simulink library "csthl20_lib"  (R2022a)
settings: Solver=VariableStepAuto  StartTime=0.0  StopTime=10.0  RelTol=1e-3
undefined symbols (not defined in the file or in its folder): alpha_vec_Cn0, b_ref, beta_vec_Cn0, Clbeta, Clda, Clddf, Cldr, Clp, Clr, Cm0, Cmda, Cmde, Cmdfn, Cmdfp, Cmdr, Cmq, Cn0, Cnda, Cnddf, Cndr, Cnp, Cnr, CX0, CXda, CXddf, CXde, CXdfn, CXdfp, CXdr, CYbeta, CYda, CYddf, CYdr, CZ0, CZda, CZde, CZdfn, CZdfp, CZdr, d_ref, mass, x_cg, x_ref
libraries: aerolibasang x3, aerolibconvert2 x2, shared6dof x1, aerolibatmos2 x1, aerolibobsolete x1, aerolibadyn x1
settings Model: Creator=The MathWorks, Inc.  LastModifiedBy=The MathWorks, Inc.
settings SolverCC: AlgebraicLoopSolver=TrustRegion
settings DataIOCC: ReturnWorkspaceOutputs=off
settings DebuggingCC: UnconnectedInputMsg=warning  UnconnectedOutputMsg=warning  UnconnectedLineMsg=warning  SFMachineParentedDataDiag=warning  ArithmeticOperatorsInVariantConditions=warning
settings SFSimCC: SimUseLocalCustomCode=off  CustomCodeUndefinedFunction=UseInterfaceOnly
settings RTWCC: RTWUseLocalCustomCode=off

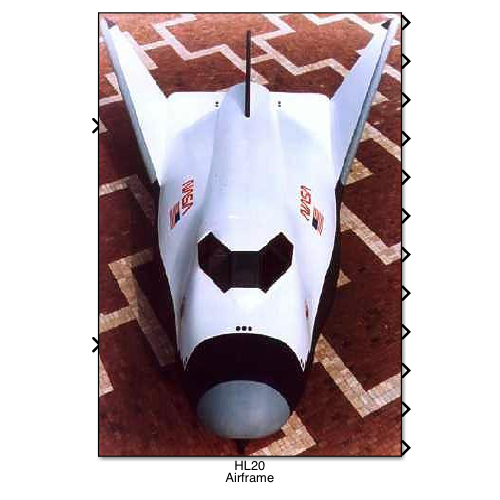
[thumbnail: Simulink's stored preview of the top-level diagram]
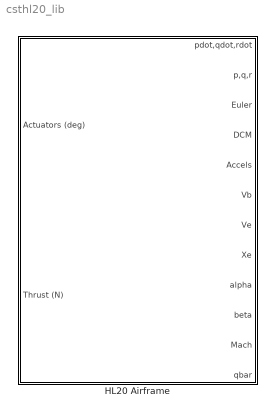
== system csthl20_lib ==
  HL20 Airframe : Subsystem
      mask Display: image('aeroblk_HL20pic.jpg')

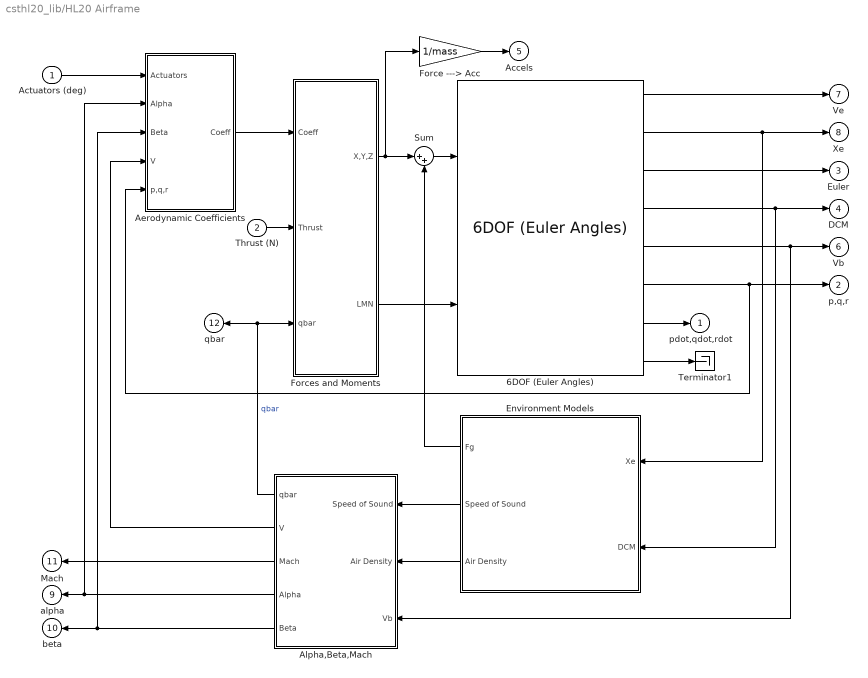
== system csthl20_lib/HL20 Airframe ==
  Actuators (deg) : Inport  Unit=deg
  Thrust (N) : Inport  Port=2  Unit=N
  6DOF (Euler Angles) : shared6dof/6DOF (Euler Angles)  units=Metric (MKS)  mtype=Fixed  rep=Euler Angles  xme_0=xme_0  Vm_0=Vmw  eul_0=Euler_0  pm_0=pm_0  mass_0=mass  mass_e=0.5  mass_f=2.0  inertia=Inertia  inertia_e=eye(3)  inertia_f=2*eye(3)  k_quat=1.0  vre_flag=on  abi_flag=off  aMode=aMode  xme_statename=''  Vm_statename=''  eul_statename=''  quat_statename=''  pm_statename=''  mass_statename=''
      settings: SourceProductBaseCode=AE,PW,DR,MT,VE
  Aerodynamic Coefficients : Subsystem
  Alpha,Beta,Mach : Subsystem
  Environment Models : Subsystem
  Force ---> Acc : Gain  Gain=1/mass  SaturateOnIntegerOverflow=on  OutDataTypeStr=Inherit: Same as input  ParamDataTypeStr=Inherit: Same as input
  Forces and Moments : Subsystem
  Sum : Sum  Inputs=|++  InputSameDT=on  SaturateOnIntegerOverflow=on  OutDataTypeStr=Inherit: Same as first input
  Terminator1 : Terminator
  pdot,qdot,rdot : Outport  Unit=rad/s^2  InitialOutput=0  VectorParamsAs1DForOutWhenUnconnected=off
  p,q,r : Outport  Port=2  Unit=rad/second  InitialOutput=0  VectorParamsAs1DForOutWhenUnconnected=off
  Euler : Outport  Port=3  Unit=rad  InitialOutput=0  VectorParamsAs1DForOutWhenUnconnected=off
  DCM : Outport  Port=4  InitialOutput=0  VectorParamsAs1DForOutWhenUnconnected=off
  Accels : Outport  Port=5  Unit=m/s^2  InitialOutput=0  VectorParamsAs1DForOutWhenUnconnected=off
  Vb : Outport  Port=6  Unit=m/second  InitialOutput=0  VectorParamsAs1DForOutWhenUnconnected=off
  Ve : Outport  Port=7  Unit=m/second  InitialOutput=0  VectorParamsAs1DForOutWhenUnconnected=off
  Xe : Outport  Port=8  Unit=meter  InitialOutput=0  VectorParamsAs1DForOutWhenUnconnected=off
  alpha : Outport  Port=9  Unit=rad  InitialOutput=0  VectorParamsAs1DForOutWhenUnconnected=off
  beta : Outport  Port=10  Unit=rad  InitialOutput=0  VectorParamsAs1DForOutWhenUnconnected=off
  Mach : Outport  Port=11  InitialOutput=0  VectorParamsAs1DForOutWhenUnconnected=off
  qbar : Outport  Port=12  Unit=Pa  InitialOutput=0  VectorParamsAs1DForOutWhenUnconnected=off
  wires:
  Alpha,Beta,Mach/5(Beta) -> beta/1, Aerodynamic Coefficients/3(Beta)
  Alpha,Beta,Mach/3(Mach) -> Mach/1
  Alpha,Beta,Mach/2(V) -> Aerodynamic Coefficients/4(V)
  Actuators (deg)/1 -> Aerodynamic Coefficients/1(Actuators)
  Force ---> Acc/1 -> Accels/1
  Environment Models/1(Fg) -> Sum/2
  Sum/1 -> 6DOF (Euler Angles)/1
  Forces and Moments/1(X,Y,Z) -> Sum/1, Force ---> Acc/1
  Alpha,Beta,Mach/1(qbar) -> qbar/1, Forces and Moments/3(qbar)  "qbar"
  Forces and Moments/2(LMN) -> 6DOF (Euler Angles)/2
  Environment Models/3(Air Density) -> Alpha,Beta,Mach/2(Air Density)
  Environment Models/2(Speed of Sound) -> Alpha,Beta,Mach/1(Speed of Sound)
  6DOF (Euler Angles)/5 -> Vb/1, Alpha,Beta,Mach/3(Vb)
  Aerodynamic Coefficients/1(Coeff) -> Forces and Moments/1(Coeff)
  Alpha,Beta,Mach/4(Alpha) -> alpha/1, Aerodynamic Coefficients/2(Alpha)
  6DOF (Euler Angles)/3 -> Euler/1
  6DOF (Euler Angles)/4 -> Environment Models/2(DCM), DCM/1
  6DOF (Euler Angles)/7 -> pdot,qdot,rdot/1
  Thrust (N)/1 -> Forces and Moments/2(Thrust)
  6DOF (Euler Angles)/6 -> p,q,r/1, Aerodynamic Coefficients/5(p,q,r)
  6DOF (Euler Angles)/2 -> Xe/1, Environment Models/1(Xe)
  6DOF (Euler Angles)/1 -> Ve/1
  6DOF (Euler Angles)/8 -> Terminator1/1

== system csthl20_lib/HL20 Airframe/Aerodynamic Coefficients ==
  Actuators : Inport
  Alpha : Inport  Port=2
  Beta : Inport  Port=3
  V : Inport  Port=4
  p,q,r : Inport  Port=5
  Actuator Increments : Subsystem
  Body Rate Damping : Subsystem
  Datum Coefficients : Subsystem
  Sum1 : Sum  Inputs=+++  InputSameDT=on  SaturateOnIntegerOverflow=on  OutDataTypeStr=Inherit: Same as first input
  alpha_rad : aerolibconvert2/Angle Conversion  IU=rad  OU=deg
  beta_rad : aerolibconvert2/Angle Conversion  IU=rad  OU=deg
  Coeff : Outport  VectorParamsAs1DForOutWhenUnconnected=off
  wires:
  Alpha/1 -> alpha_rad/1
  Beta/1 -> beta_rad/1
  alpha_rad/1 -> Body Rate Damping/3(Alpha), Datum Coefficients/1(Alpha), Actuator Increments/1(Alpha)
  p,q,r/1 -> Body Rate Damping/2(p,q,r)
  Actuators/1 -> Actuator Increments/3("Actuator Deflections ")
  Sum1/1 -> Coeff/1
  Datum Coefficients/1(cl) -> Sum1/2
  beta_rad/1 -> Datum Coefficients/2(Beta), Actuator Increments/2(Beta)
  V/1 -> Body Rate Damping/1(V)
  Body Rate Damping/1(cl) -> Sum1/1
  Actuator Increments/1(cl) -> Sum1/3

== system csthl20_lib/HL20 Airframe/Alpha,Beta,Mach ==
  note: TODO: clean up interface
  Speed of Sound : Inport
  Air Density : Inport  Port=2
  Vb : Inport  Port=3  PortDimensions=3
  Dynamic Pressure : aerolibasang/Dynamic Pressure
  "Incidence, Sideslip, & Airspeed" : aerolibasang/Incidence, Sideslip, & Airspeed
  Mach Number : aerolibasang/Mach Number
      settings: SourceProductBaseCode=AE
  qbar : Outport  Unit=Pa  InitialOutput=0  VectorParamsAs1DForOutWhenUnconnected=off
  V : Outport  Port=2  Unit=m/s  VectorParamsAs1DForOutWhenUnconnected=off
  Mach : Outport  Port=3  VectorParamsAs1DForOutWhenUnconnected=off
  Alpha : Outport  Port=4  Unit=rad  VectorParamsAs1DForOutWhenUnconnected=off
  Beta : Outport  Port=5  Unit=rad  VectorParamsAs1DForOutWhenUnconnected=off
  wires:
  Air Density/1 -> Dynamic Pressure/2
  Speed of Sound/1 -> Mach Number/2
  "Incidence, Sideslip, & Airspeed"/2 -> Beta/1  "Beta"
  "Incidence, Sideslip, & Airspeed"/3 -> V/1  "V"
  Vb/1 -> "Incidence, Sideslip, & Airspeed"/1, Mach Number/1, Dynamic Pressure/1
  "Incidence, Sideslip, & Airspeed"/1 -> Alpha/1  "Alpha"
  Mach Number/1 -> Mach/1  "Mach"
  Dynamic Pressure/1 -> qbar/1  "qbar"

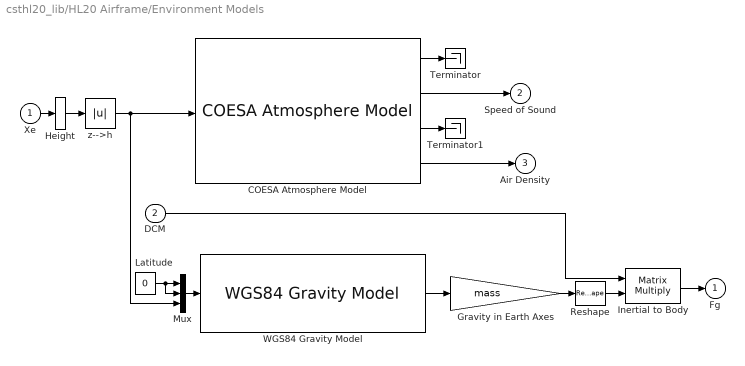
== system csthl20_lib/HL20 Airframe/Environment Models ==
  Xe : Inport  Unit=meter  PortDimensions=3
  DCM : Inport  Port=2
  COESA Atmosphere Model : aerolibatmos2/COESA Atmosphere Model  units=Metric (MKS)  spec=1976 COESA-extended U.S. Standard Atmosphere  model=Profile  profile_var=High temperature  profile_percent=10%  profile_alt=5 km (16404 ft)  envelope_var=High temperature  envelope_percent=1%  action=None
  Gravity in Earth Axes : Gain  Gain=mass  SaturateOnIntegerOverflow=on  OutDataTypeStr=Inherit: Same as input  ParamDataTypeStr=Inherit: Same as input
  Height : Selector  InputPortWidth=3  IndexOptions=Index vector (dialog)  Indices=[3]  OutputSizes=1
  Inertial to Body : Product  Multiplication=Matrix(*)  InputSameDT=on  SaturateOnIntegerOverflow=on  OutDataTypeStr=Inherit: Same as first input
  Latitude : Constant  Value=0
  Mux : Mux  Inputs=3
  Reshape : Reshape
  Terminator : Terminator
  Terminator1 : Terminator
  "WGS84 Gravity Model " : aerolibobsolete/WGS84 Gravity Model   model=WGS84 Taylor Series  units=Metric (MKS)  no_atmos=on  precessing=on  jd_loc=off  month=October  day=10  year=2004  no_centrifugal=on  action=None
      settings: SourceProductBaseCode=AE
  z-->h : Abs
  Fg : Outport  Unit=N  InitialOutput=0  VectorParamsAs1DForOutWhenUnconnected=off
  Speed of Sound : Outport  Port=2  Unit=m/second  InitialOutput=0  VectorParamsAs1DForOutWhenUnconnected=off
  Air Density : Outport  Port=3  Unit=kg/m^3  InitialOutput=0  VectorParamsAs1DForOutWhenUnconnected=off
  wires:
  "WGS84 Gravity Model "/1 -> Gravity in Earth Axes/1
  Inertial to Body/1 -> Fg/1
  DCM/1 -> Inertial to Body/1
  Gravity in Earth Axes/1 -> Reshape/1
  Latitude/1 -> Mux/1, Mux/2
  Xe/1 -> Height/1
  Height/1 -> z-->h/1
  COESA Atmosphere Model/1 -> Terminator/1
  COESA Atmosphere Model/3 -> Terminator1/1
  COESA Atmosphere Model/2 -> Speed of Sound/1
  COESA Atmosphere Model/4 -> Air Density/1
  z-->h/1 -> COESA Atmosphere Model/1, Mux/3
  Mux/1 -> "WGS84 Gravity Model "/1
  Reshape/1 -> Inertial to Body/2

== system csthl20_lib/HL20 Airframe/Forces and Moments ==
  Coeff : Inport
  Thrust : Inport  Port=2  Unit=N
  qbar : Inport  Port=3  Unit=Pa
  Aerodynamic Forces and Moments : aerolibadyn/Aerodynamic Forces and Moments   inputAxes=Body  outputForceAxes=Body  outputMomentAxes=Body  S=S_ref  b=b_ref  cbar=d_ref
  Center of Gravity : Constant  Value=[-x_cg 0 0]
  Center of Pressure : Constant  Value=[- x_ref 0 0]
  Sum : Sum  Inputs=++|  InputSameDT=on  SaturateOnIntegerOverflow=on  OutDataTypeStr=Inherit: Same as first input
  X,Y,Z : Outport  Unit=N  InitialOutput=0  VectorParamsAs1DForOutWhenUnconnected=off
  LMN : Outport  Port=2  Unit=N*m  InitialOutput=0  VectorParamsAs1DForOutWhenUnconnected=off
  wires:
  Coeff/1 -> Aerodynamic Forces and Moments/1
  qbar/1 -> Aerodynamic Forces and Moments/2
  Thrust/1 -> Sum/1
  Sum/1 -> X,Y,Z/1
  Aerodynamic Forces and Moments/2 -> LMN/1
  Aerodynamic Forces and Moments/1 -> Sum/2
  Center of Gravity/1 -> Aerodynamic Forces and Moments/3
  Center of Pressure/1 -> Aerodynamic Forces and Moments/4

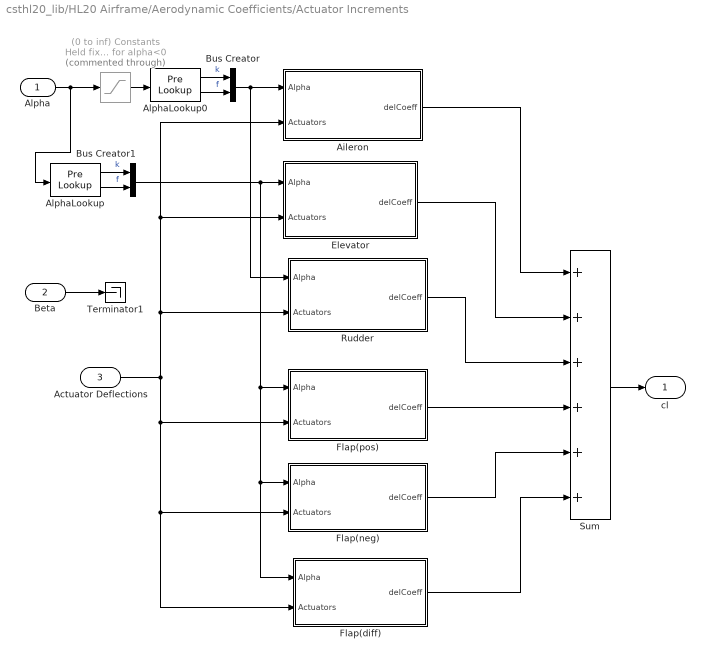
== system csthl20_lib/HL20 Airframe/Aerodynamic Coefficients/Actuator Increments ==
  Alpha : Inport
  Beta : Inport  Port=2
  "Actuator Deflections " : Inport  Port=3
  (0 to inf) Constants Held fixed for alpha<0 : Saturate  Commented=through  UpperLimit=inf  LowerLimit=0
  Aileron : Subsystem
  AlphaLookup : PreLookup  BreakpointsData=alpha_vec_0  BeginIndexSearchUsingPreviousIndexResult=on  ExtrapMethod=Linear
  AlphaLookup0 : PreLookup  BreakpointsData=alpha_vec_0  BeginIndexSearchUsingPreviousIndexResult=on  ExtrapMethod=Linear
  Bus Creator : BusCreator  Inputs=2
  Bus Creator1 : BusCreator  Inputs=2
  Elevator : Subsystem
  Flap(diff) : Subsystem
  Flap(neg) : Subsystem
  Flap(pos) : Subsystem
  Rudder : Subsystem
  Sum : Sum  Inputs=++++++  InputSameDT=on  SaturateOnIntegerOverflow=on  OutDataTypeStr=Inherit: Same as first input
  Terminator1 : Terminator
  cl : Outport  InitialOutput=0  VectorParamsAs1DForOutWhenUnconnected=off
  wires:
  Bus Creator/1 -> Aileron/1(Alpha), Rudder/1(Alpha)
  (0 to inf) Constants Held fixed for alpha<0/1 -> AlphaLookup0/1
  "Actuator Deflections "/1 -> Aileron/2(Actuators), Elevator/2(Actuators), Rudder/2(Actuators), Flap(pos)/2(Actuators), Flap(neg)/2(Actuators), Flap(diff)/2(Actuators)
  Alpha/1 -> (0 to inf) Constants Held fixed for alpha<0/1, AlphaLookup/1
  Beta/1 -> Terminator1/1
  Aileron/1(delCoeff) -> Sum/1
  Elevator/1(delCoeff) -> Sum/2
  Rudder/1(delCoeff) -> Sum/3
  Flap(pos)/1(delCoeff) -> Sum/4
  Flap(neg)/1(delCoeff) -> Sum/5
  Flap(diff)/1(delCoeff) -> Sum/6
  Sum/1 -> cl/1
  Bus Creator1/1 -> Flap(diff)/1(Alpha), Flap(neg)/1(Alpha), Flap(pos)/1(Alpha), Elevator/1(Alpha)
  AlphaLookup0/1 -> Bus Creator/1  "k"
  AlphaLookup0/2 -> Bus Creator/2  "f"
  AlphaLookup/1 -> Bus Creator1/1  "k"
  AlphaLookup/2 -> Bus Creator1/2  "f"

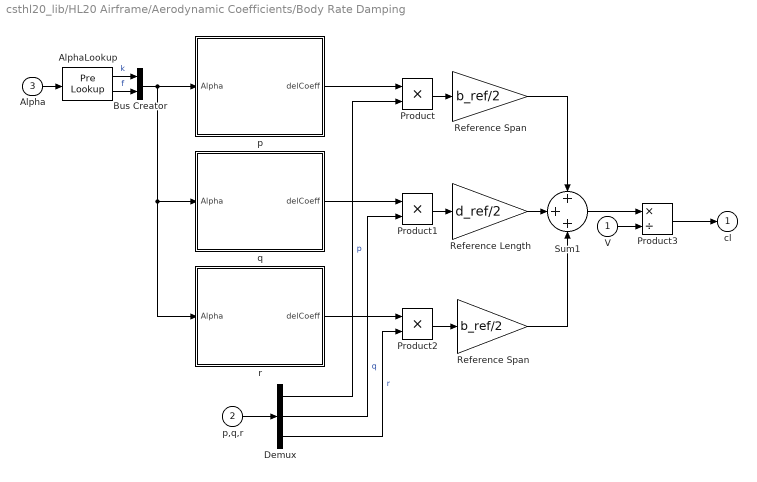
== system csthl20_lib/HL20 Airframe/Aerodynamic Coefficients/Body Rate Damping ==
  V : Inport
  p,q,r : Inport  Port=2
  Alpha : Inport  Port=3
  AlphaLookup : PreLookup  BreakpointsData=alpha_vec_damping  BeginIndexSearchUsingPreviousIndexResult=on  ExtrapMethod=Linear
  Bus Creator : BusCreator  Inputs=2
  Demux : Demux  Outputs=3
      settings: DisplayOption=none
  Product : Product  InputSameDT=on  SaturateOnIntegerOverflow=on  OutDataTypeStr=Inherit: Same as first input
  Product1 : Product  InputSameDT=on  SaturateOnIntegerOverflow=on  OutDataTypeStr=Inherit: Same as first input
  Product2 : Product  InputSameDT=on  SaturateOnIntegerOverflow=on  OutDataTypeStr=Inherit: Same as first input
  Product3 : Product  Inputs=*/  InputSameDT=on  SaturateOnIntegerOverflow=on  OutDataTypeStr=Inherit: Same as first input
  Reference Length : Gain  Gain=d_ref/2  SaturateOnIntegerOverflow=on  OutDataTypeStr=Inherit: Same as input  ParamDataTypeStr=Inherit: Same as input
  Reference Span : Gain  Gain=b_ref/2  SaturateOnIntegerOverflow=on  OutDataTypeStr=Inherit: Same as input  ParamDataTypeStr=Inherit: Same as input
  "Reference Span " : Gain  Gain=b_ref/2  SaturateOnIntegerOverflow=on  OutDataTypeStr=Inherit: Same as input  ParamDataTypeStr=Inherit: Same as input
  Sum1 : Sum  Inputs=+++  InputSameDT=on  SaturateOnIntegerOverflow=on  OutDataTypeStr=Inherit: Same as first input
  p : Subsystem
  q : Subsystem
  r : Subsystem
  cl : Outport  InitialOutput=0  VectorParamsAs1DForOutWhenUnconnected=off
  wires:
  Alpha/1 -> AlphaLookup/1
  p/1(delCoeff) -> Product/1
  q/1(delCoeff) -> Product1/1
  p,q,r/1 -> Demux/1
  Demux/1 -> Product/2  "p"
  Demux/2 -> Product1/2  "q"
  Demux/3 -> Product2/2  "r"
  Sum1/1 -> Product3/1
  V/1 -> Product3/2
  Product3/1 -> cl/1
  Product1/1 -> Reference Length/1
  Product2/1 -> "Reference Span "/1
  Product/1 -> Reference Span/1
  r/1(delCoeff) -> Product2/1
  Bus Creator/1 -> r/1(Alpha), q/1(Alpha), p/1(Alpha)
  Reference Length/1 -> Sum1/2
  Reference Span/1 -> Sum1/1
  "Reference Span "/1 -> Sum1/3
  AlphaLookup/1 -> Bus Creator/1  "k"
  AlphaLookup/2 -> Bus Creator/2  "f"

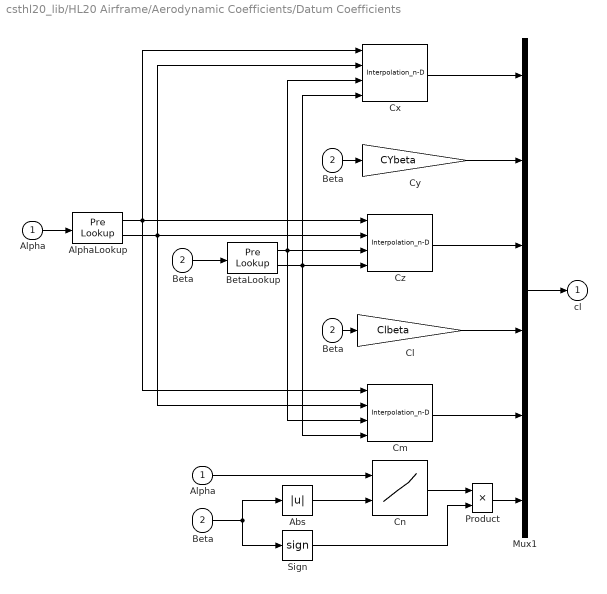
== system csthl20_lib/HL20 Airframe/Aerodynamic Coefficients/Datum Coefficients ==
  Alpha : Inport
  Beta : Inport  Port=2
  " Cn" : Lookup_n-D  BreakpointsForDimension1=alpha_vec_Cn0  BreakpointsForDimension2=beta_vec_Cn0  Table=Cn0  InternalRulePriority=Speed  RndMeth=Simplest
      settings: InputPortMap=u0,u1
  " Beta" : InportShadow  Port=2
  " Beta " : InportShadow  Port=2
  Abs : Abs
  "Alpha " : InportShadow
  AlphaLookup : PreLookup  BreakpointsData=alpha_vec_0  BeginIndexSearchUsingPreviousIndexResult=on  ExtrapMethod=Linear
  "Beta " : InportShadow  Port=2
  BetaLookup : PreLookup  BreakpointsData=beta_vec_0  BeginIndexSearchUsingPreviousIndexResult=on  ExtrapMethod=Linear
  Cl : Gain  Gain=Clbeta  SaturateOnIntegerOverflow=on  OutDataTypeStr=Inherit: Same as input  ParamDataTypeStr=Inherit: Same as input
  Cm : Interpolation_n-D  Table=Cm0'  RemoveProtectionIndex=on  SaturateOnIntegerOverflow=on
  Cx : Interpolation_n-D  Table=CX0'  RemoveProtectionIndex=on  SaturateOnIntegerOverflow=on
  Cy : Gain  Gain=CYbeta  SaturateOnIntegerOverflow=on  OutDataTypeStr=Inherit: Same as input  ParamDataTypeStr=Inherit: Same as input
  Cz : Interpolation_n-D  Table=CZ0'  RemoveProtectionIndex=on  SaturateOnIntegerOverflow=on
  Mux1 : Mux  Inputs=6
  Product : Product  InputSameDT=on  SaturateOnIntegerOverflow=on  OutDataTypeStr=Inherit: Same as first input
  Sign : Signum
  cl : Outport  InitialOutput=0  VectorParamsAs1DForOutWhenUnconnected=off
  wires:
  Sign/1 -> Product/2
  " Cn"/1 -> Product/1
  Product/1 -> Mux1/6
  Abs/1 -> " Cn"/2
  Mux1/1 -> cl/1
  Cx/1 -> Mux1/1
  Cz/1 -> Mux1/3
  Cm/1 -> Mux1/5
  Cy/1 -> Mux1/2
  Cl/1 -> Mux1/4
  Alpha/1 -> AlphaLookup/1
  Beta/1 -> BetaLookup/1
  AlphaLookup/1 -> Cx/1, Cz/1, Cm/1
  BetaLookup/1 -> Cz/3, Cx/3, Cm/3
  AlphaLookup/2 -> Cx/2, Cm/2, Cz/2
  "Beta "/1 -> Cy/1
  "Alpha "/1 -> " Cn"/1
  " Beta"/1 -> Abs/1, Sign/1
  " Beta "/1 -> Cl/1
  BetaLookup/2 -> Cz/4, Cx/4, Cm/4

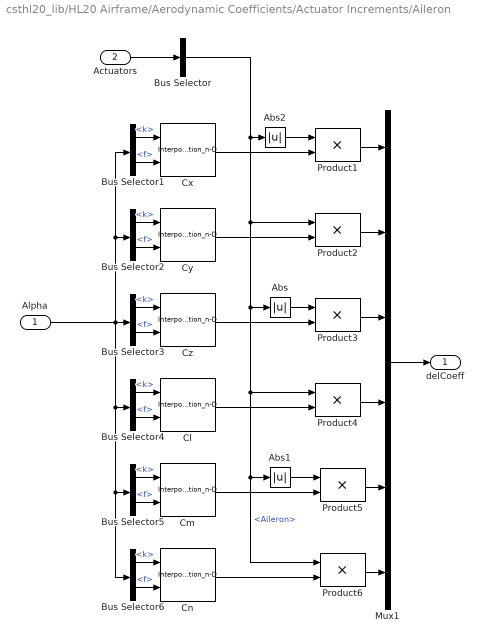
== system csthl20_lib/HL20 Airframe/Aerodynamic Coefficients/Actuator Increments/Aileron ==
  Alpha : Inport
  Actuators : Inport  Port=2
  Abs : Abs
  Abs1 : Abs
  Abs2 : Abs
  Bus Selector : BusSelector  OutputSignals=Aileron
  Bus Selector{1..6} (6 alike) : BusSelector  OutputSignals=k,f
  Cl : Interpolation_n-D  NumberOfTableDimensions=1  Table=Clda  RemoveProtectionIndex=on  SaturateOnIntegerOverflow=on
      settings: InputPortMap=u0,u1
  Cm : Interpolation_n-D  NumberOfTableDimensions=1  Table=Cmda  RemoveProtectionIndex=on  SaturateOnIntegerOverflow=on
      settings: InputPortMap=u0,u1
  Cn : Interpolation_n-D  NumberOfTableDimensions=1  Table=Cnda  RemoveProtectionIndex=on  SaturateOnIntegerOverflow=on
      settings: InputPortMap=u0,u1
  Cx : Interpolation_n-D  NumberOfTableDimensions=1  Table=CXda  RemoveProtectionIndex=on  SaturateOnIntegerOverflow=on
      settings: InputPortMap=u0,u1
  Cy : Interpolation_n-D  NumberOfTableDimensions=1  Table=CYda  RemoveProtectionIndex=on  SaturateOnIntegerOverflow=on
      settings: InputPortMap=u0,u1
  Cz : Interpolation_n-D  NumberOfTableDimensions=1  Table=CZda  RemoveProtectionIndex=on  SaturateOnIntegerOverflow=on
      settings: InputPortMap=u0,u1
  Mux1 : Mux  Inputs=6
  Product{1..6} (6 alike) : Product  InputSameDT=on  SaturateOnIntegerOverflow=on  OutDataTypeStr=Inherit: Same as first input
  delCoeff : Outport  VectorParamsAs1DForOutWhenUnconnected=off
  wires:
  Actuators/1 -> Bus Selector/1
  Mux1/1 -> delCoeff/1
  Product1/1 -> Mux1/1
  Cx/1 -> Product1/2
  Product2/1 -> Mux1/2
  Cy/1 -> Product2/2
  Product3/1 -> Mux1/3
  Cz/1 -> Product3/2
  Cl/1 -> Product4/2
  Product4/1 -> Mux1/4
  Cm/1 -> Product5/2
  Product5/1 -> Mux1/5
  Cn/1 -> Product6/2
  Product6/1 -> Mux1/6
  Bus Selector/1 -> Product6/1, Abs1/1, Product4/1, Abs/1, Product2/1, Abs2/1  "<Aileron>"
  Abs/1 -> Product3/1
  Abs1/1 -> Product5/1
  Abs2/1 -> Product1/1
  Alpha/1 -> Bus Selector1/1, Bus Selector2/1, Bus Selector5/1, Bus Selector6/1, Bus Selector4/1, Bus Selector3/1
  Bus Selector1/1 -> Cx/1  "<k>"
  Bus Selector1/2 -> Cx/2  "<f>"
  Bus Selector2/1 -> Cy/1  "<k>"
  Bus Selector2/2 -> Cy/2  "<f>"
  Bus Selector3/1 -> Cz/1  "<k>"
  Bus Selector3/2 -> Cz/2  "<f>"
  Bus Selector4/1 -> Cl/1  "<k>"
  Bus Selector4/2 -> Cl/2  "<f>"
  Bus Selector5/1 -> Cm/1  "<k>"
  Bus Selector5/2 -> Cm/2  "<f>"
  Bus Selector6/1 -> Cn/1  "<k>"
  Bus Selector6/2 -> Cn/2  "<f>"

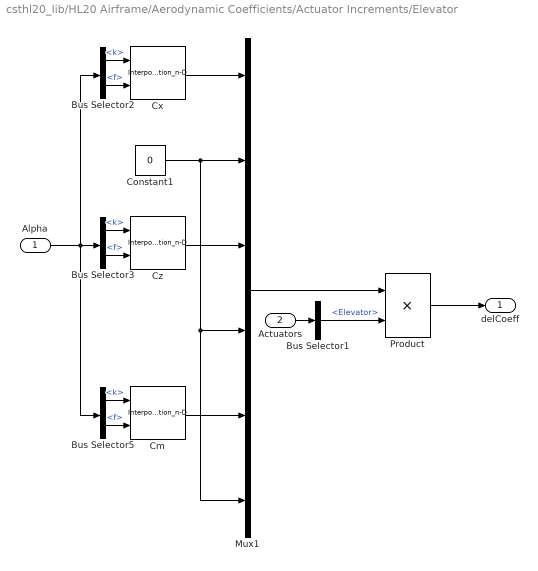
== system csthl20_lib/HL20 Airframe/Aerodynamic Coefficients/Actuator Increments/Elevator ==
  Alpha : Inport
  Actuators : Inport  Port=2
  Bus Selector1 : BusSelector  OutputSignals=Elevator
  Bus Selector2 : BusSelector  OutputSignals=k,f
  Bus Selector3 : BusSelector  OutputSignals=k,f
  Bus Selector5 : BusSelector  OutputSignals=k,f
  Cm : Interpolation_n-D  NumberOfTableDimensions=1  Table=Cmde  RemoveProtectionIndex=on  SaturateOnIntegerOverflow=on
      settings: InputPortMap=u0,u1
  Constant1 : Constant  Value=0
  Cx : Interpolation_n-D  NumberOfTableDimensions=1  Table=CXde  RemoveProtectionIndex=on  SaturateOnIntegerOverflow=on
      settings: InputPortMap=u0,u1
  Cz : Interpolation_n-D  NumberOfTableDimensions=1  Table=CZde  RemoveProtectionIndex=on  SaturateOnIntegerOverflow=on
      settings: InputPortMap=u0,u1
  Mux1 : Mux  Inputs=6
  Product : Product  InputSameDT=on  SaturateOnIntegerOverflow=on  OutDataTypeStr=Inherit: Same as first input
  delCoeff : Outport  VectorParamsAs1DForOutWhenUnconnected=off
  wires:
  Product/1 -> delCoeff/1
  Mux1/1 -> Product/1
  Alpha/1 -> Bus Selector2/1, Bus Selector3/1, Bus Selector5/1
  Cx/1 -> Mux1/1
  Cz/1 -> Mux1/3
  Cm/1 -> Mux1/5
  Constant1/1 -> Mux1/2, Mux1/4, Mux1/6
  Actuators/1 -> Bus Selector1/1
  Bus Selector1/1 -> Product/2  "<Elevator>"
  Bus Selector2/1 -> Cx/1  "<k>"
  Bus Selector2/2 -> Cx/2  "<f>"
  Bus Selector3/1 -> Cz/1  "<k>"
  Bus Selector3/2 -> Cz/2  "<f>"
  Bus Selector5/1 -> Cm/1  "<k>"
  Bus Selector5/2 -> Cm/2  "<f>"

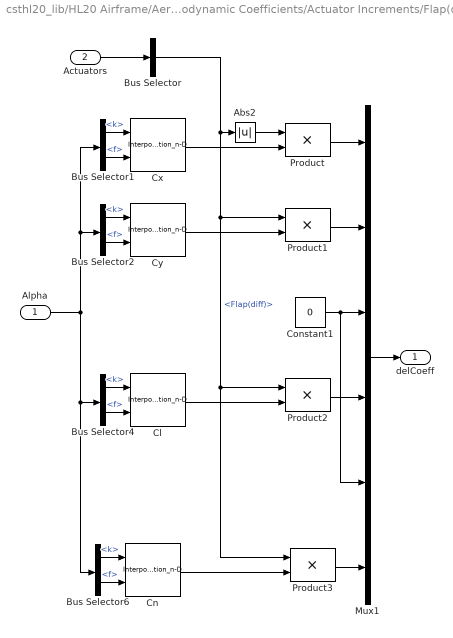
== system csthl20_lib/HL20 Airframe/Aerodynamic Coefficients/Actuator Increments/Flap(diff) ==
  Alpha : Inport
  Actuators : Inport  Port=2
  Abs2 : Abs
  Bus Selector : BusSelector  OutputSignals=Flap(diff)
  Bus Selector{1..2,4,6} (4 alike) : BusSelector  OutputSignals=k,f
  Cl : Interpolation_n-D  NumberOfTableDimensions=1  Table=Clddf  RemoveProtectionIndex=on  SaturateOnIntegerOverflow=on
      settings: InputPortMap=u0,u1
  Cn : Interpolation_n-D  NumberOfTableDimensions=1  Table=Cnddf  RemoveProtectionIndex=on  SaturateOnIntegerOverflow=on
      settings: InputPortMap=u0,u1
  Constant1 : Constant  Value=0
  Cx : Interpolation_n-D  NumberOfTableDimensions=1  Table=CXddf  RemoveProtectionIndex=on  SaturateOnIntegerOverflow=on
      settings: InputPortMap=u0,u1
  Cy : Interpolation_n-D  NumberOfTableDimensions=1  Table=CYddf  RemoveProtectionIndex=on  SaturateOnIntegerOverflow=on
      settings: InputPortMap=u0,u1
  Mux1 : Mux  Inputs=6
  Product{,1..3} (4 alike) : Product  InputSameDT=on  SaturateOnIntegerOverflow=on  OutDataTypeStr=Inherit: Same as first input
  delCoeff : Outport  VectorParamsAs1DForOutWhenUnconnected=off
  wires:
  Mux1/1 -> delCoeff/1
  Alpha/1 -> Bus Selector4/1, Bus Selector6/1, Bus Selector1/1, Bus Selector2/1
  Actuators/1 -> Bus Selector/1
  Product/1 -> Mux1/1
  Cx/1 -> Product/2
  Bus Selector/1 -> Product3/1, Product2/1, Product1/1, Abs2/1  "<Flap(diff)>"
  Product1/1 -> Mux1/2
  Product2/1 -> Mux1/4
  Cl/1 -> Product2/2
  Cy/1 -> Product1/2
  Product3/1 -> Mux1/6
  Cn/1 -> Product3/2
  Abs2/1 -> Product/1
  Constant1/1 -> Mux1/3, Mux1/5
  Bus Selector1/1 -> Cx/1  "<k>"
  Bus Selector1/2 -> Cx/2  "<f>"
  Bus Selector2/1 -> Cy/1  "<k>"
  Bus Selector2/2 -> Cy/2  "<f>"
  Bus Selector4/1 -> Cl/1  "<k>"
  Bus Selector4/2 -> Cl/2  "<f>"
  Bus Selector6/1 -> Cn/1  "<k>"
  Bus Selector6/2 -> Cn/2  "<f>"

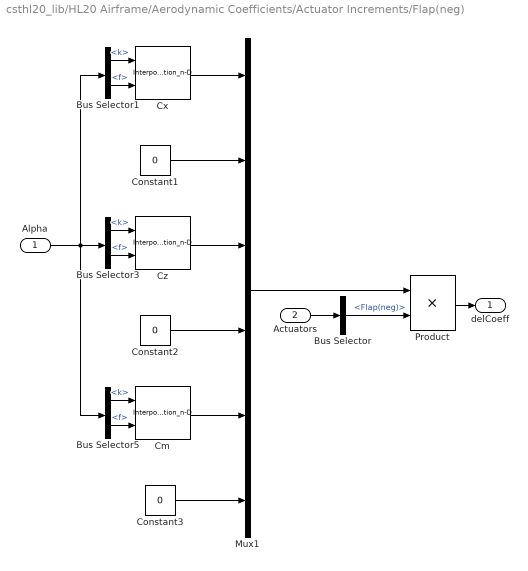
== system csthl20_lib/HL20 Airframe/Aerodynamic Coefficients/Actuator Increments/Flap(neg) ==
  Alpha : Inport
  Actuators : Inport  Port=2
  Bus Selector : BusSelector  OutputSignals=Flap(neg)
  Bus Selector1 : BusSelector  OutputSignals=k,f
  Bus Selector3 : BusSelector  OutputSignals=k,f
  Bus Selector5 : BusSelector  OutputSignals=k,f
  Cm : Interpolation_n-D  NumberOfTableDimensions=1  Table=Cmdfn  RemoveProtectionIndex=on  SaturateOnIntegerOverflow=on
      settings: InputPortMap=u0,u1
  Constant1 : Constant  Value=0
  Constant2 : Constant  Value=0
  Constant3 : Constant  Value=0
  Cx : Interpolation_n-D  NumberOfTableDimensions=1  Table=CXdfn  RemoveProtectionIndex=on  SaturateOnIntegerOverflow=on
      settings: InputPortMap=u0,u1
  Cz : Interpolation_n-D  NumberOfTableDimensions=1  Table=CZdfn  RemoveProtectionIndex=on  SaturateOnIntegerOverflow=on
      settings: InputPortMap=u0,u1
  Mux1 : Mux  Inputs=6
  Product : Product  InputSameDT=on  SaturateOnIntegerOverflow=on  OutDataTypeStr=Inherit: Same as first input
  delCoeff : Outport  VectorParamsAs1DForOutWhenUnconnected=off
  wires:
  Cm/1 -> Mux1/5
  Cz/1 -> Mux1/3
  Cx/1 -> Mux1/1
  Alpha/1 -> Bus Selector5/1, Bus Selector3/1, Bus Selector1/1
  Mux1/1 -> Product/1
  Product/1 -> delCoeff/1
  Actuators/1 -> Bus Selector/1
  Constant1/1 -> Mux1/2
  Constant2/1 -> Mux1/4
  Constant3/1 -> Mux1/6
  Bus Selector/1 -> Product/2  "<Flap(neg)>"
  Bus Selector5/1 -> Cm/1  "<k>"
  Bus Selector5/2 -> Cm/2  "<f>"
  Bus Selector3/1 -> Cz/1  "<k>"
  Bus Selector3/2 -> Cz/2  "<f>"
  Bus Selector1/1 -> Cx/1  "<k>"
  Bus Selector1/2 -> Cx/2  "<f>"

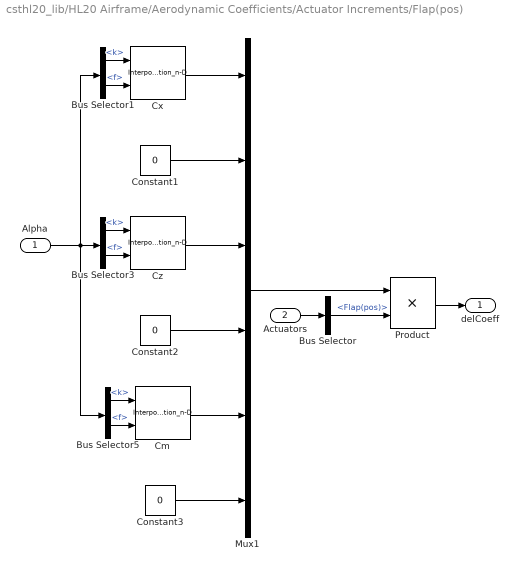
== system csthl20_lib/HL20 Airframe/Aerodynamic Coefficients/Actuator Increments/Flap(pos) ==
  Alpha : Inport
  Actuators : Inport  Port=2
  Bus Selector : BusSelector  OutputSignals=Flap(pos)
  Bus Selector1 : BusSelector  OutputSignals=k,f
  Bus Selector3 : BusSelector  OutputSignals=k,f
  Bus Selector5 : BusSelector  OutputSignals=k,f
  Cm : Interpolation_n-D  NumberOfTableDimensions=1  Table=Cmdfp  RemoveProtectionIndex=on  SaturateOnIntegerOverflow=on
      settings: InputPortMap=u0,u1
  Constant1 : Constant  Value=0
  Constant2 : Constant  Value=0
  Constant3 : Constant  Value=0
  Cx : Interpolation_n-D  NumberOfTableDimensions=1  Table=CXdfp  RemoveProtectionIndex=on  SaturateOnIntegerOverflow=on
      settings: InputPortMap=u0,u1
  Cz : Interpolation_n-D  NumberOfTableDimensions=1  Table=CZdfp  RemoveProtectionIndex=on  SaturateOnIntegerOverflow=on
      settings: InputPortMap=u0,u1
  Mux1 : Mux  Inputs=6
  Product : Product  InputSameDT=on  SaturateOnIntegerOverflow=on  OutDataTypeStr=Inherit: Same as first input
  delCoeff : Outport  VectorParamsAs1DForOutWhenUnconnected=off
  wires:
  Product/1 -> delCoeff/1
  Mux1/1 -> Product/1
  Alpha/1 -> Bus Selector5/1, Bus Selector3/1, Bus Selector1/1
  Cx/1 -> Mux1/1
  Cz/1 -> Mux1/3
  Cm/1 -> Mux1/5
  Constant1/1 -> Mux1/2
  Constant2/1 -> Mux1/4
  Constant3/1 -> Mux1/6
  Actuators/1 -> Bus Selector/1
  Bus Selector/1 -> Product/2  "<Flap(pos)>"
  Bus Selector5/1 -> Cm/1  "<k>"
  Bus Selector5/2 -> Cm/2  "<f>"
  Bus Selector3/1 -> Cz/1  "<k>"
  Bus Selector3/2 -> Cz/2  "<f>"
  Bus Selector1/1 -> Cx/1  "<k>"
  Bus Selector1/2 -> Cx/2  "<f>"

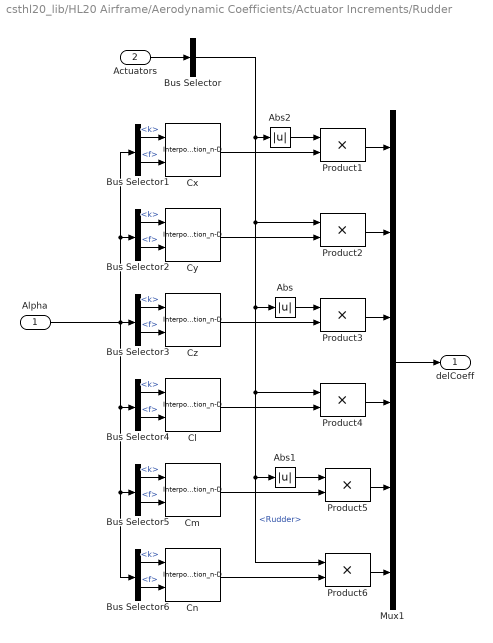
== system csthl20_lib/HL20 Airframe/Aerodynamic Coefficients/Actuator Increments/Rudder ==
  Alpha : Inport
  Actuators : Inport  Port=2
  Abs : Abs
  Abs1 : Abs
  Abs2 : Abs
  Bus Selector : BusSelector  OutputSignals=Rudder
  Bus Selector{1..6} (6 alike) : BusSelector  OutputSignals=k,f
  Cl : Interpolation_n-D  NumberOfTableDimensions=1  Table=Cldr  RemoveProtectionIndex=on  SaturateOnIntegerOverflow=on
      settings: InputPortMap=u0,u1
  Cm : Interpolation_n-D  NumberOfTableDimensions=1  Table=Cmdr  RemoveProtectionIndex=on  SaturateOnIntegerOverflow=on
      settings: InputPortMap=u0,u1
  Cn : Interpolation_n-D  NumberOfTableDimensions=1  Table=Cndr  RemoveProtectionIndex=on  SaturateOnIntegerOverflow=on
      settings: InputPortMap=u0,u1
  Cx : Interpolation_n-D  NumberOfTableDimensions=1  Table=CXdr  RemoveProtectionIndex=on  SaturateOnIntegerOverflow=on
      settings: InputPortMap=u0,u1
  Cy : Interpolation_n-D  NumberOfTableDimensions=1  Table=CYdr  RemoveProtectionIndex=on  SaturateOnIntegerOverflow=on
      settings: InputPortMap=u0,u1
  Cz : Interpolation_n-D  NumberOfTableDimensions=1  Table=CZdr  RemoveProtectionIndex=on  SaturateOnIntegerOverflow=on
      settings: InputPortMap=u0,u1
  Mux1 : Mux  Inputs=6
  Product{1..6} (6 alike) : Product  InputSameDT=on  SaturateOnIntegerOverflow=on  OutDataTypeStr=Inherit: Same as first input
  delCoeff : Outport  VectorParamsAs1DForOutWhenUnconnected=off
  wires:
  Actuators/1 -> Bus Selector/1
  Mux1/1 -> delCoeff/1
  Product1/1 -> Mux1/1
  Cx/1 -> Product1/2
  Product2/1 -> Mux1/2
  Cy/1 -> Product2/2
  Product3/1 -> Mux1/3
  Cz/1 -> Product3/2
  Cl/1 -> Product4/2
  Product4/1 -> Mux1/4
  Cm/1 -> Product5/2
  Product5/1 -> Mux1/5
  Cn/1 -> Product6/2
  Product6/1 -> Mux1/6
  Bus Selector/1 -> Abs2/1, Product2/1, Abs/1, Product4/1, Abs1/1, Product6/1  "<Rudder>"
  Abs/1 -> Product3/1
  Abs1/1 -> Product5/1
  Abs2/1 -> Product1/1
  Alpha/1 -> Bus Selector3/1, Bus Selector4/1, Bus Selector6/1, Bus Selector5/1, Bus Selector2/1, Bus Selector1/1
  Bus Selector1/1 -> Cx/1  "<k>"
  Bus Selector1/2 -> Cx/2  "<f>"
  Bus Selector2/1 -> Cy/1  "<k>"
  Bus Selector2/2 -> Cy/2  "<f>"
  Bus Selector3/1 -> Cz/1  "<k>"
  Bus Selector3/2 -> Cz/2  "<f>"
  Bus Selector4/1 -> Cl/1  "<k>"
  Bus Selector4/2 -> Cl/2  "<f>"
  Bus Selector5/1 -> Cm/1  "<k>"
  Bus Selector5/2 -> Cm/2  "<f>"
  Bus Selector6/1 -> Cn/1  "<k>"
  Bus Selector6/2 -> Cn/2  "<f>"

== system csthl20_lib/HL20 Airframe/Aerodynamic Coefficients/Body Rate Damping/p ==
  Alpha : Inport
  Bus Selector : BusSelector  OutputSignals=k,f
  Bus Selector1 : BusSelector  OutputSignals=k,f
  Cl : Interpolation_n-D  NumberOfTableDimensions=1  Table=Clp  RemoveProtectionIndex=on  SaturateOnIntegerOverflow=on
      settings: InputPortMap=u0,u1
  Cn : Interpolation_n-D  NumberOfTableDimensions=1  Table=Cnp  RemoveProtectionIndex=on  SaturateOnIntegerOverflow=on
      settings: InputPortMap=u0,u1
  Constant1 : Constant  Value=0
  Mux1 : Mux  Inputs=6
  delCoeff : Outport  VectorParamsAs1DForOutWhenUnconnected=off
  wires:
  Mux1/1 -> delCoeff/1
  Constant1/1 -> Mux1/1, Mux1/5, Mux1/3, Mux1/2  "Cxp"
  Cn/1 -> Mux1/6
  Cl/1 -> Mux1/4  "Cl"
  Alpha/1 -> Bus Selector/1, Bus Selector1/1
  Bus Selector/1 -> Cl/1  "<k>"
  Bus Selector/2 -> Cl/2  "<f>"
  Bus Selector1/1 -> Cn/1  "<k>"
  Bus Selector1/2 -> Cn/2  "<f>"

== system csthl20_lib/HL20 Airframe/Aerodynamic Coefficients/Body Rate Damping/q ==
  Alpha : Inport
  Bus Selector1 : BusSelector  OutputSignals=k,f
  Cmq : Interpolation_n-D  NumberOfTableDimensions=1  Table=Cmq  RemoveProtectionIndex=on  SaturateOnIntegerOverflow=on
      settings: InputPortMap=u0,u1
  Constant3 : Constant  Value=0
  Mux1 : Mux  Inputs=6
  delCoeff : Outport  VectorParamsAs1DForOutWhenUnconnected=off
  wires:
  Cmq/1 -> Mux1/5
  Constant3/1 -> Mux1/1, Mux1/2, Mux1/3, Mux1/6, Mux1/4
  Mux1/1 -> delCoeff/1
  Alpha/1 -> Bus Selector1/1
  Bus Selector1/1 -> Cmq/1  "<k>"
  Bus Selector1/2 -> Cmq/2  "<f>"

== system csthl20_lib/HL20 Airframe/Aerodynamic Coefficients/Body Rate Damping/r ==
  Alpha : Inport
  Bus Selector : BusSelector  OutputSignals=k,f
  Bus Selector1 : BusSelector  OutputSignals=k,f
  Cl : Interpolation_n-D  NumberOfTableDimensions=1  Table=Clr  RemoveProtectionIndex=on  SaturateOnIntegerOverflow=on
      settings: InputPortMap=u0,u1
  Cn : Interpolation_n-D  NumberOfTableDimensions=1  Table=Cnr  RemoveProtectionIndex=on  SaturateOnIntegerOverflow=on
      settings: InputPortMap=u0,u1
  Constant : Constant  Value=0
  Mux1 : Mux  Inputs=6
  delCoeff : Outport  VectorParamsAs1DForOutWhenUnconnected=off
  wires:
  Cn/1 -> Mux1/6
  Cl/1 -> Mux1/4  "Cl"
  Constant/1 -> Mux1/1, Mux1/2, Mux1/5, Mux1/3  "Cxr"
  Mux1/1 -> delCoeff/1
  Alpha/1 -> Bus Selector1/1, Bus Selector/1
  Bus Selector/1 -> Cl/1  "<k>"
  Bus Selector/2 -> Cl/2  "<f>"
  Bus Selector1/1 -> Cn/1  "<k>"
  Bus Selector1/2 -> Cn/2  "<f>"
